simulink model "model_1b_IPV"  (R2019b)
settings: Solver=VariableStepAuto  StartTime=0.0  StopTime=10.0  RelTol=1e-3
values from neighbouring files (symbols this model uses):
  deltat = sample_time    (= 0.004)    [params.m]
  Kc = pi.Kc    [params.m]
  sample_time = 1/5*wn    (= 0.004)    [params.m]
  step_amplitude = 67    [params.m]
  tauI = pi.tauI    [params.m]
  Umax = 1    [params.m]
  Umin = 0    [params.m]
libraries: arduinolib x2
settings Model: Creator=adityaaaap  LastModifiedBy=adityaaaap

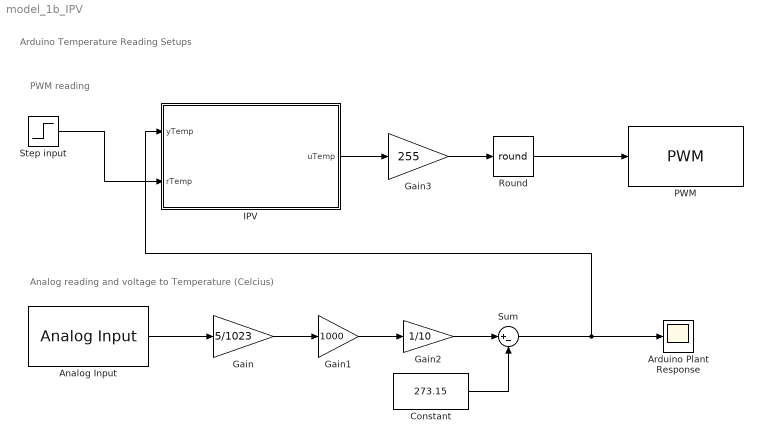
== system model_1b_IPV ==
  note: Analog reading and voltage to Temperature (Celcius)
  note: Arduino Temperature Reading Setups
  note: PWM reading
  Analog Input : arduinolib/Analog Input  pinNumber=0  ReadResultsOnly=off  ConversionTriggerSource=Software  ExternalTriggerType=uint32(0)  OutputDataType=uint16  EnableConversionCompleteNotify=off  EnableOuputStatus=off  SampleTime=1  blockPlatform=arduino
  Arduino Plant Response : Scope
  Constant : Constant  Value=273.15
  Gain : Gain  Gain=5/1023
  Gain1 : Gain  Gain=1000
  Gain2 : Gain  Gain=1/10
  Gain3 : Gain  Gain=255
  "IPV " : MATLAB Function  TreatAsAtomicUnit=on
  PWM : arduinolib/PWM  pinNumber=7  EnableInputFrequency=off  InitialFrequency=2000  InitialDutyCycle=0  NotificationType=None  blockPlatform=arduino
  "Round " : Rounding  Operator=round
  Step input : Step  Time=0  After=step_amplitude  SampleTime=sample_time
  Sum : Sum  Inputs=|+-
  wires:
  "Round "/1 -> PWM/1
  Analog Input/1 -> Gain/1
  Gain/1 -> Gain1/1
  Gain2/1 -> Sum/1
  Gain3/1 -> "Round "/1
  Constant/1 -> Sum/2
  Gain1/1 -> Gain2/1
  Sum/1 -> "IPV "/1(yTemp), Arduino Plant Response/1
  Step input/1 -> "IPV "/2(rTemp)
  "IPV "/1(uTemp) -> Gain3/1

== matlab function model_1b_IPV/IPV  ==
  settings: updateMethod=DISCRETE  sampleTime=deltat
  data: yTemp input; uTemp output; rTemp input; Kc parameter; tauI parameter; deltat parameter; Umin parameter; Umax parameter
function uTemp = IPV(yTemp,rTemp,Kc, tauI, deltat, Umin, Umax)
    persistent uPast 
    if isempty(uPast)
        uPast=0;
    end
    
    persistent yPast 
    if isempty(yPast)
        yPast=0; 
    end
    
    persistent uDPast 
    if isempty(uDPast)
        uDPast=0;
    end
    
    persistent rPast 
    if isempty(rPast)
        rPast=0;
    end
   
    uTemp = uPast+...
        Kc*(-yTemp+yPast)+ ...
        (Kc*deltat)/tauI*(rTemp-yTemp);

    if (uTemp>Umax) 
        uTemp=Umax;
    end
    
    if (uTemp<Umin) 
        uTemp=Umin; 
    end
    
    uPast=uTemp; 
    yPast=yTemp; 
    rPast=rTemp;
end
